simulink model "Open_Loop_Flight_Log_Simulation"  (R2023b)
settings: Solver=FixedStepAuto  StartTime=0.0  StopTime=10.899  FixedStep=0.01  RelTol=1e-3
values from neighbouring files (symbols this model uses):
  controller = controller.addGain(aptos, steadyState, velocity)    [parameter_uncertainty.m]    (also in robustness_analysis.m = controller.addGain(nominal, steadyState, velocity); simulator.m; simulator_multi_sim.m; state_space_formulation_velocity_varying.m)
undefined symbols (not defined in the file or in its folder): pitchAngle, pitchRate, rollAngle, rollRate, time, velocitySmooth, yawAngle, yawRate
libraries: simulink_extras x20
settings Model: Creator=mn19ty  LastModifiedBy=sambr
settings DataIOCC: ReturnWorkspaceOutputsName=yout
settings ModelReferenceCC: EnableRefExpFcnMdlSchedulingChecks=on

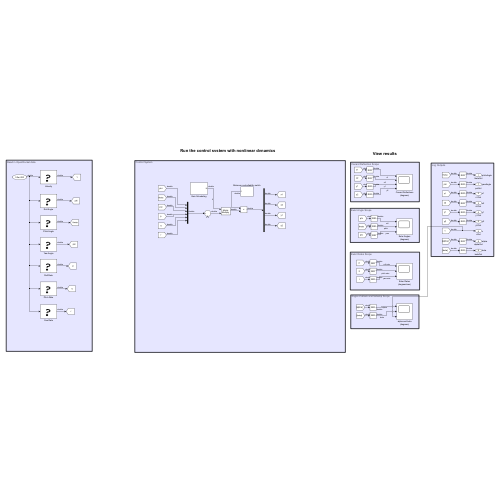
[thumbnail: Simulink's stored preview of the top-level diagram]
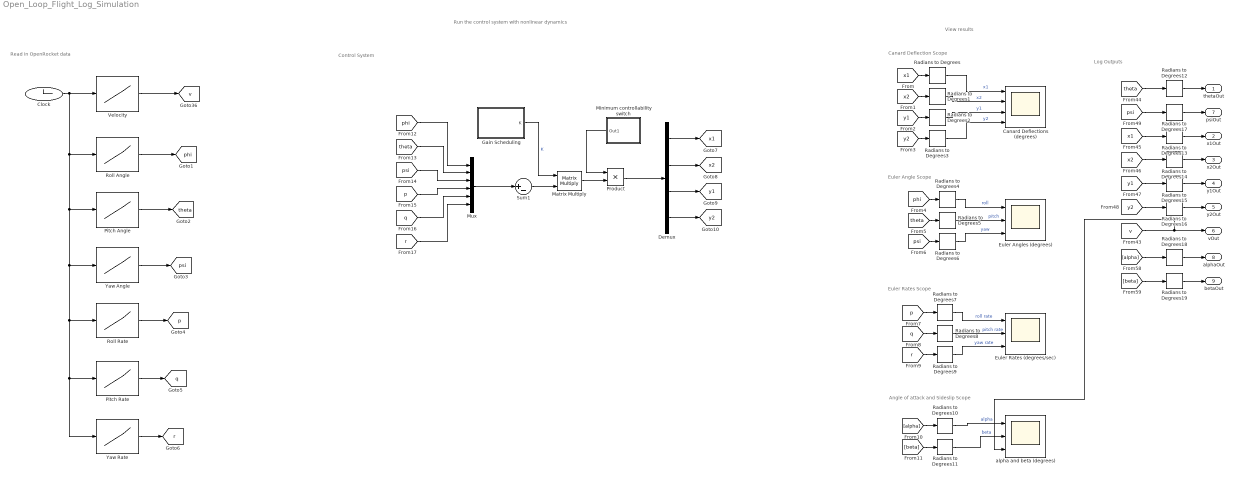
== system Open_Loop_Flight_Log_Simulation ==
  note: Log Outputs
  note: Read in OpenRocket data
  note: Angle of attack and Sideslip Scope
  note: View results
  note: Run the control system with nonlinear dynamics
  note: Euler Rates Scope
  note: Euler Angle Scope
  note: Canard Deflection Scope
  note: Control System
  Canard Deflections (degrees) : Scope  NumInputPorts=4
  Clock : Clock
  Demux : Demux
  Euler Angles (degrees) : Scope  NumInputPorts=3
  Euler Rates (degrees/sec) : Scope  NumInputPorts=3
  Gain Scheduling : Subsystem
  Matrix Multiply : Product  Multiplication=Matrix(*)
  Minimum controllability switch : Subsystem
  Mux : Mux  Inputs=6
  Pitch Angle : Lookup_n-D  NumberOfTableDimensions=1  BreakpointsForDimension1=time  Table=pitchAngle  InternalRulePriority=Speed  RndMeth=Simplest
  Pitch Rate : Lookup_n-D  NumberOfTableDimensions=1  BreakpointsForDimension1=time  Table=pitchRate  InternalRulePriority=Speed  RndMeth=Simplest
  Product : Product
  Radians to Degrees{,1..19} (20 alike) : simulink_extras/Transformations/Radians to Degrees
  Roll Angle : Lookup_n-D  NumberOfTableDimensions=1  BreakpointsForDimension1=time  Table=rollAngle  InternalRulePriority=Speed  RndMeth=Simplest
  Roll Rate : Lookup_n-D  NumberOfTableDimensions=1  BreakpointsForDimension1=time  Table=rollRate  InternalRulePriority=Speed  RndMeth=Simplest
  Sum1 : Sum  Inputs=|+-
  Velocity : Lookup_n-D  NumberOfTableDimensions=1  BreakpointsForDimension1=time  Table=velocitySmooth  InternalRulePriority=Speed  RndMeth=Simplest
  Yaw Angle : Lookup_n-D  NumberOfTableDimensions=1  BreakpointsForDimension1=time  Table=yawAngle  InternalRulePriority=Speed  RndMeth=Simplest
  Yaw Rate : Lookup_n-D  NumberOfTableDimensions=1  BreakpointsForDimension1=time  Table=yawRate  InternalRulePriority=Speed  RndMeth=Simplest
  alpha and beta (degrees) : Scope  NumInputPorts=3
  thetaOut : Outport  SignalName=pitchAngle
  x1Out : Outport  Port=2  SignalName=x1
  x2Out : Outport  Port=3  SignalName=x2
  y1Out : Outport  Port=4  SignalName=y1
  y2Out : Outport  Port=5  SignalName=y2
  vOut : Outport  Port=6  SignalName=v
  psiOut : Outport  Port=7  SignalName=yawAngle
  alphaOut : Outport  Port=8  SignalName=alpha
  betaOut : Outport  Port=9  SignalName=beta
  tag scope: p=global, phi=global, psi=global, q=global, r=global, theta=global, v=global, x1=global, x2=global, y1=global, y2=global
  wires:
  [x1] -> Radians to Degrees/1
  [y1] -> Radians to Degrees2/1
  [x2] -> Radians to Degrees1/1
  [y2] -> Radians to Degrees3/1
  [theta] -> Radians to Degrees5/1
  [phi] -> Radians to Degrees4/1
  [psi] -> Radians to Degrees6/1
  [q] -> Radians to Degrees8/1
  [p] -> Radians to Degrees7/1
  [r] -> Radians to Degrees9/1
  [alpha] -> Radians to Degrees10/1
  [beta] -> Radians to Degrees11/1
  Sum1/1 -> Matrix Multiply/2
  [phi] -> Mux/1
  [theta] -> Mux/2
  [p] -> Mux/4
  [q] -> Mux/5
  [psi] -> Mux/3
  [r] -> Mux/6
  Mux/1 -> Sum1/1
  Radians to Degrees/1 -> Canard Deflections (degrees)/1  "x1"
  Radians to Degrees1/1 -> Canard Deflections (degrees)/2  "x2"
  Radians to Degrees2/1 -> Canard Deflections (degrees)/3  "y1"
  Radians to Degrees3/1 -> Canard Deflections (degrees)/4  "y2"
  Radians to Degrees4/1 -> Euler Angles (degrees)/1  "roll"
  Radians to Degrees5/1 -> Euler Angles (degrees)/2  "pitch"
  Radians to Degrees6/1 -> Euler Angles (degrees)/3  "yaw"
  Radians to Degrees7/1 -> Euler Rates (degrees/sec)/1  "roll rate"
  Radians to Degrees8/1 -> Euler Rates (degrees/sec)/2  "pitch rate"
  Radians to Degrees9/1 -> Euler Rates (degrees/sec)/3  "yaw rate"
  Radians to Degrees10/1 -> alpha and beta (degrees)/1  "alpha"
  Radians to Degrees11/1 -> alpha and beta (degrees)/2  "beta"
  Clock/1 -> Yaw Rate/1, Pitch Rate/1, Roll Rate/1, Yaw Angle/1, Pitch Angle/1, Roll Angle/1, Velocity/1
  [theta] -> Radians to Degrees12/1
  Radians to Degrees12/1 -> thetaOut/1
  [x1] -> Radians to Degrees13/1
  Radians to Degrees13/1 -> x1Out/1
  [x2] -> Radians to Degrees14/1
  Radians to Degrees14/1 -> x2Out/1
  Radians to Degrees15/1 -> y1Out/1
  [y1] -> Radians to Degrees15/1
  [y2] -> Radians to Degrees16/1
  Radians to Degrees16/1 -> y2Out/1
  Gain Scheduling/1(K) -> Matrix Multiply/1  "K"
  Minimum controllability switch/1(Out1) -> Product/1
  Matrix Multiply/1 -> Product/2
  Product/1 -> Demux/1
  [v] -> alpha and beta (degrees)/3, vOut/1
  Radians to Degrees17/1 -> psiOut/1
  [psi] -> Radians to Degrees17/1
  Radians to Degrees18/1 -> alphaOut/1
  [alpha] -> Radians to Degrees18/1
  [beta] -> Radians to Degrees19/1
  Radians to Degrees19/1 -> betaOut/1
  Velocity/1 -> [v]
  Yaw Rate/1 -> [r]
  Pitch Rate/1 -> [q]
  Roll Rate/1 -> [p]
  Yaw Angle/1 -> [psi]
  Pitch Angle/1 -> [theta]
  Roll Angle/1 -> [phi]
  Demux/1 -> [x1]
  Demux/2 -> [x2]
  Demux/3 -> [y1]
  Demux/4 -> [y2]

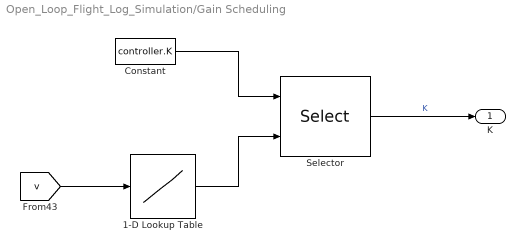
== system Open_Loop_Flight_Log_Simulation/Gain Scheduling ==
  1-D Lookup Table : Lookup_n-D  NumberOfTableDimensions=1  BreakpointsForDimension1=controller.velocities  Table=1:length(controller.velocities)  InterpMethod=Nearest  InternalRulePriority=Speed  OutDataTypeStr=int8  RndMeth=Simplest
  Constant : Constant  Value=controller.K
  Selector : Selector  NumberOfDimensions=3  InputPortWidth=3  IndexOptions=Select all,Select all,Index vector (port)  Indices=[1 3],1,1  OutputSizes=1,1,1
  K : Outport
  wires:
  [v] -> 1-D Lookup Table/1
  Selector/1 -> K/1  "K"
  1-D Lookup Table/1 -> Selector/2
  Constant/1 -> Selector/1

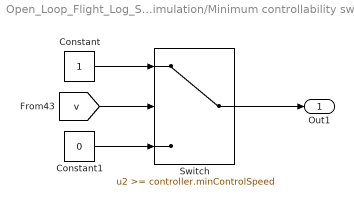
== system Open_Loop_Flight_Log_Simulation/Minimum controllability switch ==
  Constant : Constant
  Constant1 : Constant  Value=0
  Switch : Switch  Threshold=controller.minControlSpeed  SaturateOnIntegerOverflow=off  InputSameDT=off
  Out1 : Outport
  wires:
  [v] -> Switch/2
  Switch/1 -> Out1/1
  Constant/1 -> Switch/1
  Constant1/1 -> Switch/3
